simulink model "VAJA3"  (R2020a)
settings: Solver=VariableStepAuto  StartTime=0.0  StopTime=15000  RelTol=1e-3
values from neighbouring files (symbols this model uses):
  a = -(lambda * S) / (m * cp * d)    [AVS_4in5.m]    (also in Simulink.m = a/2)
  b = 1 / (m * cp)    (= 1.64690382082e-05)    [AVS_4in5.m]    (also in Matlab_AVS.m; Simulink.m)
settings Model: Creator=Jaka  LastModifiedBy=Jaka

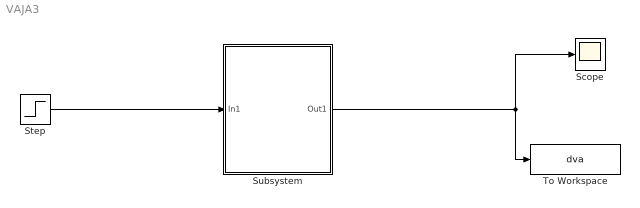
== system VAJA3 ==
  Scope : Scope
  Step : Step  Time=10000  After=500  SampleTime=1
  Subsystem : Subsystem
  To Workspace : ToWorkspace  VariableName=dva  SampleTime=-1
  wires:
  Subsystem/1(Out1) -> To Workspace/1, Scope/1
  Step/1 -> Subsystem/1(In1)

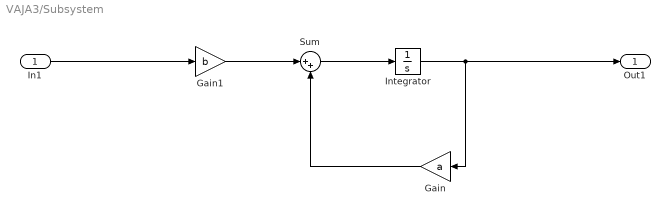
== system VAJA3/Subsystem ==
  In1 : Inport
  Gain : Gain  Gain=a
  Gain1 : Gain  Gain=b
  Integrator : Integrator  InitialCondition=-5
  Sum : Sum  Inputs=|++
  Out1 : Outport
  wires:
  Integrator/1 -> Out1/1, Gain/1
  In1/1 -> Gain1/1
  Sum/1 -> Integrator/1
  Gain/1 -> Sum/2
  Gain1/1 -> Sum/1
